simulink model "mconversion12a"  (Simulink 6.0)
settings: Solver=FixedStepDiscrete  StartTime=0.0  StopTime=2  FixedStep=1  RelTol=1e-3
libraries: mconversion12aLib2 x1, mconversion12aLib1 x1
settings Model: Creator=mshakeri  LastModifiedBy=awarlock  ExtModeAutoUpdateStatusClock=off
settings DataIOCC: ExternalInput=utStr  SaveFormat=StructureWithTime  SaveState=on  SignalLoggingName=logsOut
settings OptimizationCC: InlineParams=on  InlineInvariantSignals=off  LifeSpan=1
settings DebuggingCC: CheckExecutionContextPreStartOutputMsg=on  CheckExecutionContextRuntimeOutputMsg=on  SolverPrmCheckMsg=none
settings HardwareCC: TargetUnknown=on
settings RTWCC: SystemTargetFile=ert.tlc  TemplateMakefile=ert_default_tmf  RetainRTWFile=on  ProcessScript=ert_make_rtw_hook
settings ERTTargetCC: TargetFcnLib=ansi_tfl_tmw.mat  GenFloatMathFcnCalls=ANSI_C  GenerateSampleERTMain=on  SupportContinuousTime=on  SupportNonInlinedSFcns=on  RootIOFormat=Individual Arguments  ERTCustomFileTemplate=example_file_process.tlc  InitialValueSource=Model
settings SFSimCC: SFSimApplyToAllLibs=on  SFSimBuildMode=Incremental

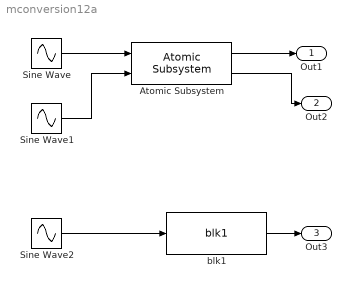
== system mconversion12a ==
  Atomic Subsystem : mconversion12aLib2/Atomic Subsystem
  Sine Wave : Sin  SampleTime=0
  Sine Wave1 : Sin  SampleTime=0
  Sine Wave2 : Sin  SampleTime=0
  blk1 : mconversion12aLib1/blk1
  Out1 : Outport
  Out2 : Outport  Port=2
  Out3 : Outport  Port=3
  wires:
  Sine Wave/1 -> Atomic Subsystem/1
  Sine Wave1/1 -> Atomic Subsystem/2
  Atomic Subsystem/1 -> Out1/1
  Atomic Subsystem/2 -> Out2/1
  Sine Wave2/1 -> blk1/1
  blk1/1 -> Out3/1
